simulink model "ChallengeMPC"  (R2020b)
settings: Solver=VariableStepAuto  StartTime=0.0  StopTime=86400  RelTol=1e-3
undefined symbols (not defined in the file): A_OBS, Aa, Ac, B_OBS, Ba, Bc, C_OBS, Ca, Cc, D_OBS, Dc, F, H, lambdae, lambdau, Np, Te
settings Model: Creator=jack  LastModifiedBy=ouyang

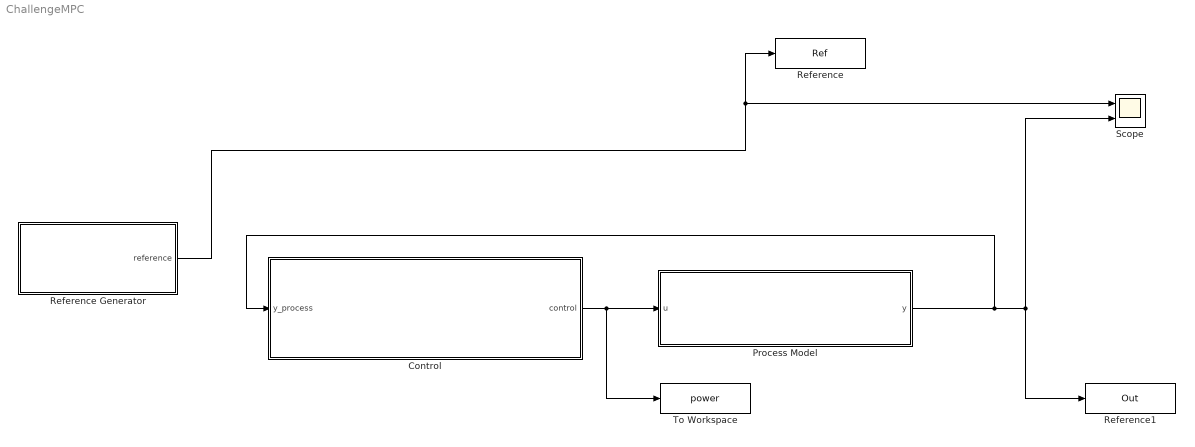
== system ChallengeMPC ==
  Control : Subsystem
  Process Model : Subsystem
  Reference : ToWorkspace  VariableName=Ref  SaveFormat=Timeseries  SampleTime=-1
  Reference Generator : Subsystem
  Reference1 : ToWorkspace  VariableName=Out  SaveFormat=Timeseries  SampleTime=-1
  Scope : Scope  NumInputPorts=2
  To Workspace : ToWorkspace  VariableName=power  SaveFormat=Timeseries  SampleTime=-1
  wires:
  Reference Generator/1(reference) -> Reference/1, Scope/1
  Control/1(control) -> To Workspace/1, Process Model/1(u)
  Process Model/1(y) -> Control/1(y_process), Scope/2, Reference1/1

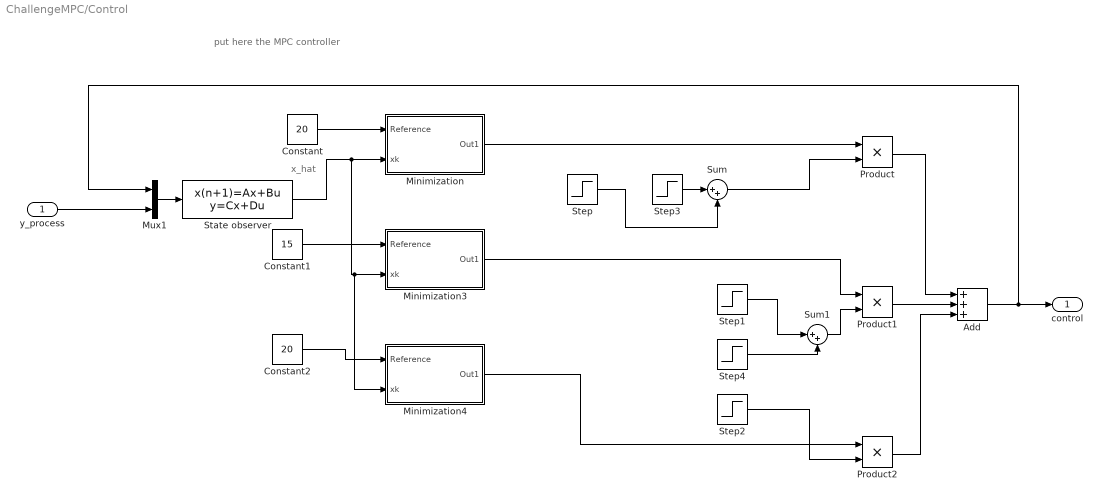
== system ChallengeMPC/Control ==
  note: x_hat
  note: put here the MPC controller
  y_process : Inport
  Add : Sum  Inputs=+++
  Constant : Constant  Value=20
  Constant1 : Constant  Value=15
  Constant2 : Constant  Value=20
  Minimization : Subsystem
  Minimization3 : Subsystem
  Minimization4 : Subsystem
  Mux1 : Mux  Inputs=2
  Product : Product
  Product1 : Product
  Product2 : Product
  State observer : DiscreteStateSpace  A=A_OBS  B=B_OBS  C=C_OBS  D=D_OBS  SampleTime=Te
  Step : Step  Time=32400  After=0  SampleTime=0
  Step1 : Step  Time=0  After=0  SampleTime=1
  Step2 : Step  Time=57600  SampleTime=0
  Step3 : Step  Time=0  After=0  SampleTime=0
  Step4 : Step  Time=0  After=0  SampleTime=0
  Sum : Sum  Inputs=|++
  Sum1 : Sum  Inputs=|++
  control : Outport
  wires:
  State observer/1 -> Minimization4/2(xk), Minimization3/2(xk), Minimization/2(xk)
  Mux1/1 -> State observer/1
  y_process/1 -> Mux1/2
  Constant/1 -> Minimization/1(Reference)
  Step3/1 -> Sum/1
  Step4/1 -> Sum1/2
  Add/1 -> Mux1/1, control/1
  Step/1 -> Sum/2
  Step1/1 -> Sum1/1
  Minimization/1(Out1) -> Product/1
  Sum/1 -> Product/2
  Product/1 -> Add/1
  Sum1/1 -> Product1/2
  Minimization3/1(Out1) -> Product1/1
  Product1/1 -> Add/2
  Step2/1 -> Product2/2
  Minimization4/1(Out1) -> Product2/1
  Product2/1 -> Add/3
  Constant1/1 -> Minimization3/1(Reference)
  Constant2/1 -> Minimization4/1(Reference)

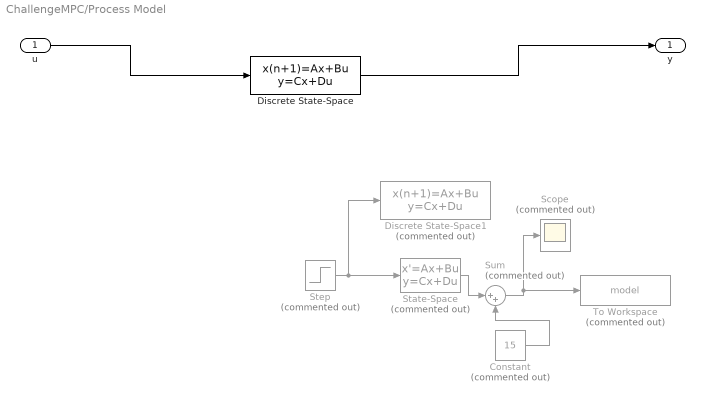
== system ChallengeMPC/Process Model ==
  u : Inport
  Constant : Constant  Commented=on  Value=15
  Discrete State-Space : DiscreteStateSpace  A=Aa  B=Ba  C=Ca  D=zeros(1,1)  InitialCondition=[0;0;0;0;0;15]  SampleTime=Te
  Discrete State-Space1 : DiscreteStateSpace  Commented=on  A=Aa  B=Ba  C=Ca  D=zeros(1,1)  InitialCondition=[0;0;0;0;0;15]  SampleTime=Te
  Scope : Scope  Commented=on
  State-Space : StateSpace  Commented=on  A=Ac  B=Bc  C=Cc  D=Dc  InitialCondition=0
  Step : Step  Commented=on  Time=1000  Before=1  After=0  SampleTime=0
  Sum : Sum  Commented=on  Inputs=|++
  To Workspace : ToWorkspace  Commented=on  VariableName=model  SaveFormat=Timeseries  SampleTime=-1
  y : Outport
  wires:
  u/1 -> Discrete State-Space/1
  Discrete State-Space/1 -> y/1
  Step/1 -> Discrete State-Space1/1, State-Space/1
  Constant/1 -> Sum/2
  State-Space/1 -> Sum/1
  Sum/1 -> Scope/1, To Workspace/1

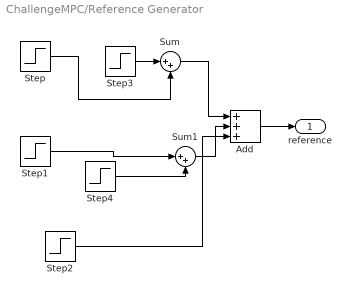
== system ChallengeMPC/Reference Generator ==
  Add : Sum  Inputs=+++
  Step : Step  Time=32400  After=-20  SampleTime=0
  Step1 : Step  Time=32400  After=15  SampleTime=0
  Step2 : Step  Time=57600  After=20  SampleTime=0
  Step3 : Step  Time=0  After=20  SampleTime=0
  Step4 : Step  Time=57600  After=-15  SampleTime=0
  Sum : Sum  Inputs=|++
  Sum1 : Sum  Inputs=|++
  reference : Outport
  wires:
  Step1/1 -> Sum1/1
  Step/1 -> Sum/2
  Add/1 -> reference/1
  Step2/1 -> Add/3
  Sum1/1 -> Add/2
  Sum/1 -> Add/1
  Step4/1 -> Sum1/2
  Step3/1 -> Sum/1

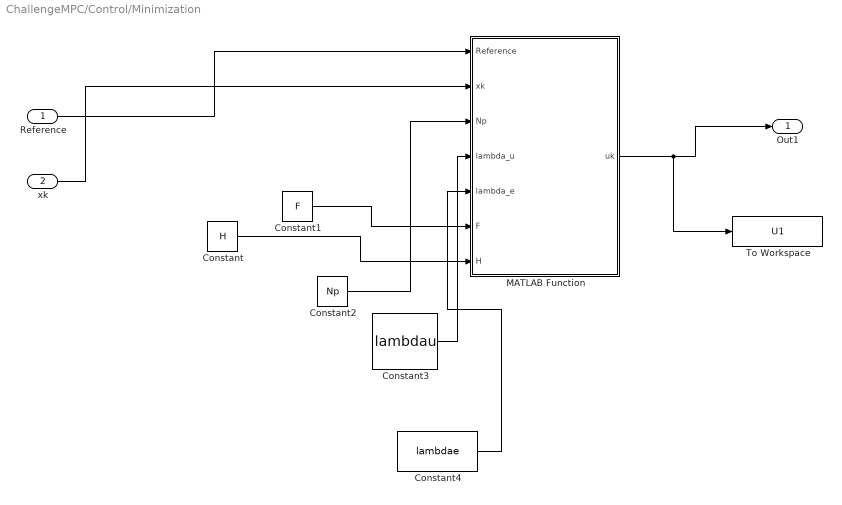
== system ChallengeMPC/Control/Minimization ==
  Reference : Inport
  xk : Inport  Port=2
  Constant : Constant  Value=H  VectorParams1D=off
  Constant1 : Constant  Value=F  VectorParams1D=off
  Constant2 : Constant  Value=Np
  Constant3 : Constant  Value=lambdau
  Constant4 : Constant  Value=lambdae
  MATLAB Function : MATLAB Function  TreatAsAtomicUnit=on
  To Workspace : ToWorkspace  VariableName=U1  SaveFormat=Timeseries  SampleTime=-1
  Out1 : Outport
  wires:
  xk/1 -> MATLAB Function/2(xk)
  Reference/1 -> MATLAB Function/1(Reference)
  MATLAB Function/1(uk) -> To Workspace/1, Out1/1
  Constant/1 -> MATLAB Function/7(H)
  Constant1/1 -> MATLAB Function/6(F)
  Constant2/1 -> MATLAB Function/3(Np)
  Constant3/1 -> MATLAB Function/4(lambda_u)
  Constant4/1 -> MATLAB Function/5(lambda_e)

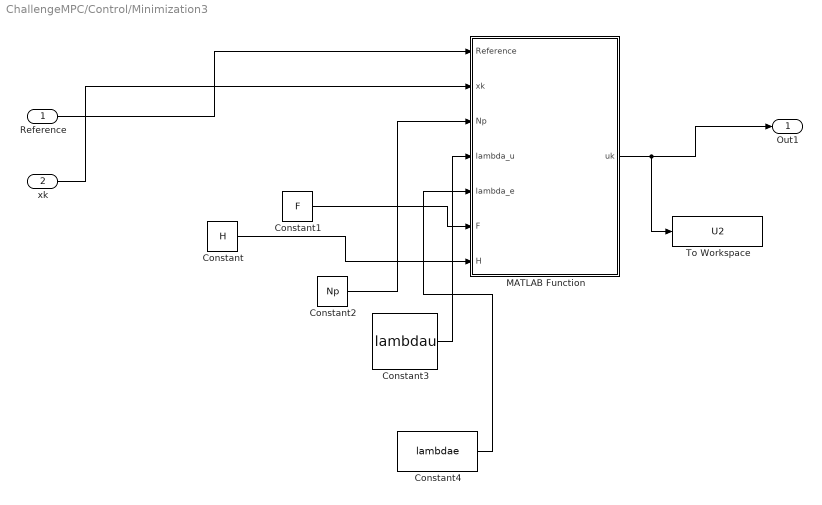
== system ChallengeMPC/Control/Minimization3 ==
  Reference : Inport
  xk : Inport  Port=2
  Constant : Constant  Value=H  VectorParams1D=off
  Constant1 : Constant  Value=F  VectorParams1D=off
  Constant2 : Constant  Value=Np
  Constant3 : Constant  Value=lambdau
  Constant4 : Constant  Value=lambdae
  MATLAB Function : MATLAB Function  TreatAsAtomicUnit=on
  To Workspace : ToWorkspace  VariableName=U2  SaveFormat=Timeseries  SampleTime=-1
  Out1 : Outport
  wires:
  xk/1 -> MATLAB Function/2(xk)
  Reference/1 -> MATLAB Function/1(Reference)
  MATLAB Function/1(uk) -> To Workspace/1, Out1/1
  Constant/1 -> MATLAB Function/7(H)
  Constant1/1 -> MATLAB Function/6(F)
  Constant2/1 -> MATLAB Function/3(Np)
  Constant3/1 -> MATLAB Function/4(lambda_u)
  Constant4/1 -> MATLAB Function/5(lambda_e)

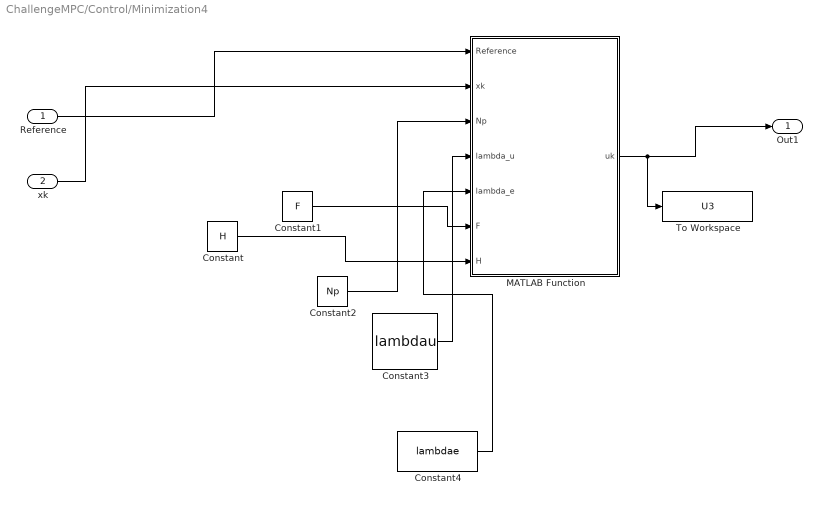
== system ChallengeMPC/Control/Minimization4 ==
  Reference : Inport
  xk : Inport  Port=2
  Constant : Constant  Value=H  VectorParams1D=off
  Constant1 : Constant  Value=F  VectorParams1D=off
  Constant2 : Constant  Value=Np
  Constant3 : Constant  Value=lambdau
  Constant4 : Constant  Value=lambdae
  MATLAB Function : MATLAB Function  TreatAsAtomicUnit=on
  To Workspace : ToWorkspace  VariableName=U3  SaveFormat=Timeseries  SampleTime=-1
  Out1 : Outport
  wires:
  xk/1 -> MATLAB Function/2(xk)
  Reference/1 -> MATLAB Function/1(Reference)
  MATLAB Function/1(uk) -> To Workspace/1, Out1/1
  Constant/1 -> MATLAB Function/7(H)
  Constant1/1 -> MATLAB Function/6(F)
  Constant2/1 -> MATLAB Function/3(Np)
  Constant3/1 -> MATLAB Function/4(lambda_u)
  Constant4/1 -> MATLAB Function/5(lambda_e)

== matlab function ChallengeMPC/Control/Minimization/MATLAB Function ==
  data: Reference input; uk output; xk input; Np input; lambda_u input; lambda_e input; F input; H input
function uk = fcn(Reference,xk,Np,lambda_u,lambda_e,F,H)

uk = 0;
coder.extrinsic('quadprog');

% define H and f in quadprog

Reference = Reference*ones(Np,1);
W = [eye(Np), zeros(Np,3*Np); zeros(Np), lambda_u*0.16*0.16*eye(Np), zeros(Np,2*Np); zeros(2*Np,2*Np), lambda_e*eye(2*Np)];
f = [-Reference', zeros(1,3*Np)];

% define A in quadprog
A = [zeros(Np), eye(Np), zeros(Np,2*Np);zeros(Np), -eye(Np), zeros(Np,2*Np)];
b = [1.5*ones(Np,1);zeros(Np,1)];
% A = [zeros(Np), eye(Np), zeros(Np,2*Np);zeros(Np), -eye(Np), zeros(Np,2*Np); eye(Np), zeros(Np,3*Np)];
% b = [1.5*ones(Np,1);zeros(Np,1); 25*ones(Np,1)];

% Aeq and beq in quadprog 
Aeq = [eye(Np), -H, zeros(Np,2*Np)];
beq = F*xk;

[Uopt] = quadprog(W,f,A,b,Aeq,beq);

Uopt;

uk = Uopt(Np+1,1);

== matlab function ChallengeMPC/Control/Minimization3/MATLAB Function ==
  data: Reference input; uk output; xk input; Np input; lambda_u input; lambda_e input; F input; H input
function uk = fcn(Reference,xk,Np,lambda_u,lambda_e,F,H)

uk = 0;
coder.extrinsic('quadprog');

% define H and f in quadprog

Reference = Reference*ones(Np,1);
W = [eye(Np), zeros(Np,3*Np); zeros(Np), lambda_u*0.18*0.18*eye(Np), zeros(Np,2*Np); zeros(2*Np,2*Np), lambda_e*eye(2*Np)];
f = [-Reference', zeros(1,3*Np)];

% define A in quadprog
A = [zeros(Np), eye(Np), zeros(Np,2*Np);zeros(Np), -eye(Np), zeros(Np,2*Np)];
b = [1.5*ones(Np,1);zeros(Np,1)];
% A = [zeros(Np), eye(Np), zeros(Np,2*Np);zeros(Np), -eye(Np), zeros(Np,2*Np); eye(Np), zeros(Np,3*Np)];
% b = [1.5*ones(Np,1);zeros(Np,1); 25*ones(Np,1)];

% Aeq and beq in quadprog 
Aeq = [eye(Np), -H, zeros(Np,2*Np)];
beq = F*xk;

[Uopt] = quadprog(W,f,A,b,Aeq,beq);

Uopt;

uk = Uopt(Np+1,1);

== matlab function ChallengeMPC/Control/Minimization4/MATLAB Function ==
  data: Reference input; uk output; xk input; Np input; lambda_u input; lambda_e input; F input; H input
function uk = fcn(Reference,xk,Np,lambda_u,lambda_e,F,H)

uk = 0;
coder.extrinsic('quadprog');

% define H and f in quadprog

Reference = Reference*ones(Np,1);
W = [eye(Np), zeros(Np,3*Np); zeros(Np), lambda_u*0.2*0.2*eye(Np), zeros(Np,2*Np); zeros(2*Np,2*Np), lambda_e*eye(2*Np)];
f = [-Reference', zeros(1,3*Np)];

% define A in quadprog
A = [zeros(Np), eye(Np), zeros(Np,2*Np);zeros(Np), -eye(Np), zeros(Np,2*Np)];
b = [1.5*ones(Np,1);zeros(Np,1)];
% A = [zeros(Np), eye(Np), zeros(Np,2*Np);zeros(Np), -eye(Np), zeros(Np,2*Np); eye(Np), zeros(Np,3*Np)];
% b = [1.5*ones(Np,1);zeros(Np,1); 25*ones(Np,1)];

% Aeq and beq in quadprog 
Aeq = [eye(Np), -H, zeros(Np,2*Np)];
beq = F*xk;

[Uopt] = quadprog(W,f,A,b,Aeq,beq);

Uopt;

uk = Uopt(Np+1,1);
